simulink model "VVA_pressure_dynamic_basefreq_sin"  (R2023b)
settings: Solver=FixedStepAuto  StartTime=0.0  StopTime=6  MaxStep=1e-3  RelTol=1e-3
values from neighbouring files (symbols this model uses):
  x = [2*10^5	3*10^5	4*10^5	5*10^5	6*10^5	7*10^5	8*10^5]    [Q.m]    (also in new_run_compare_export_jieyue.m = ts.Data(:); new_run_compare_sin_export.m = ts.Data(:); objfun_ga.m = double(x(:)); run_compare_jieyue.m = ts.Data(:))
  y = [0 ... (first row only)    [Q.m]    (also in new_run_compare_export_jieyue.m = interp1(t0u, x0u, t(:), method, 'extrap'); new_run_compare_sin_export.m = interp1(t0u, x0u, t(:), method, 'extrap'); objfun_ga.m = y(ia); run_compare_jieyue.m = interp1(t0u, x0u, t(:), method, 'extrap'))
  z = [0.893557423	1.334431826	1.76701406	2.210901891	2.65062	3.098039216	3.535707573 ... (first row only)    [Q.m]
undefined symbols (not defined in the file or in its folder): freq_mode
libraries: fuzblock x2, simulink x2
settings Model: Creator=Administrator  LastModifiedBy=47371
settings SolverCC: MaxConsecutiveMinStep=2  ZeroCrossAlgorithm=Adaptive  AlgebraicLoopSolver=TrustRegion
settings DebuggingCC: MaskedZcDiagnostic=none  IgnoredZcDiagnostic=none  ArithmeticOperatorsInVariantConditions=warning
settings SFSimCC: CustomCodeUndefinedFunction=UseInterfaceOnly

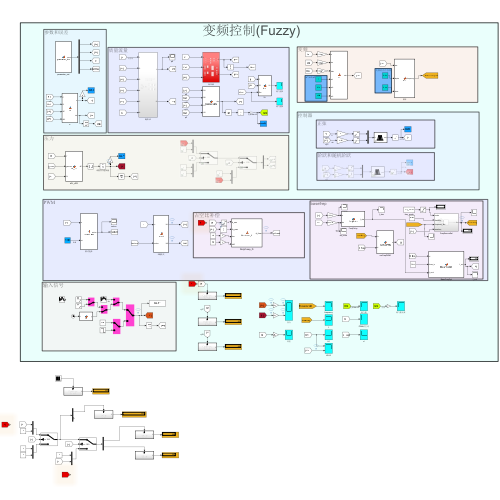
[thumbnail: Simulink's stored preview of the top-level diagram]
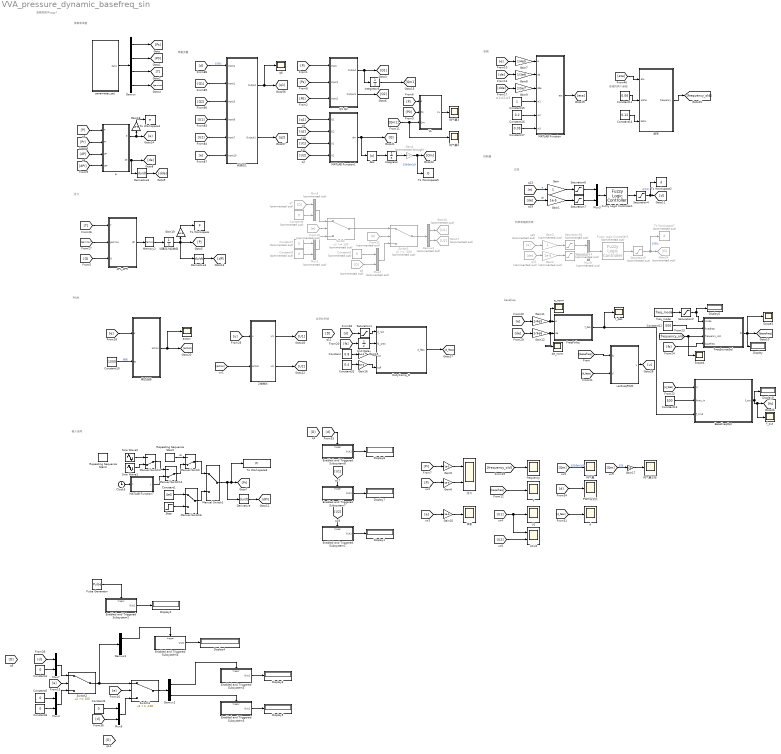
== system VVA_pressure_dynamic_basefreq_sin ==
  note: 输入信号
  note: 占空比补偿
  note: 正弦
  note: 阶跃和随机阶跃
  note: 变频控制(Fuzzy)
  note: 变频
  note: basefrep
  note: 控制器
  note: 压力
  note: 参数和误差
  note: 质量流量
  note: PWM
  note: 变频的两个参数
  note: w1,w2,w3
  2阀模式 : MATLAB Function  TreatAsAtomicUnit=on  SystemSampleTime=0.001
  Abs : Abs  SaturateOnIntegerOverflow=off
  BaseFreqOpt : MATLAB Function  TreatAsAtomicUnit=on
  Clock5 : Clock
  Constant : Constant  Value=0.8
  Constant1 : Constant  Value=4e5
  Constant10 : Constant  Value=1000
  Constant11 : Constant  Value=0.06
  Constant12 : Constant  Value=500
  Constant13 : Constant  Value=500
  Constant14 : Constant  Value=0.12
  Constant15 : Constant
  Constant16 : Constant  Value=0.2
  Constant17 : Constant  Value=0.05
  Constant{2,4..5,8} (4 alike) : Constant  Value=0
  Constant{3,6..7,9} (4 alike) : Constant  Commented=on  Value=0
  Constant32 : Constant  Value=0.4
  Demux : Demux
  Demux1 : Demux  Commented=on  Outputs=2
  Demux2 : Demux  Outputs=2
  Demux3 : Demux  Outputs=2
  Derivative : Derivative
  Derivative1 : Derivative
  Derivative2 : Derivative
  Display{,1..9} (10 alike) : Display
  DutyComp_D : MATLAB Function  TreatAsAtomicUnit=on
  Enabled and Triggered Subsystem1 : Subsystem  TreatAsAtomicUnit=on
  Enabled and Triggered Subsystem2 : Subsystem  TreatAsAtomicUnit=on
  Enabled and Triggered Subsystem3 : Subsystem  TreatAsAtomicUnit=on
  Enabled and Triggered Subsystem4 : Subsystem  TreatAsAtomicUnit=on
  Enabled and Triggered Subsystem5 : Subsystem  TreatAsAtomicUnit=on
  Enabled and Triggered Subsystem7 : Subsystem  TreatAsAtomicUnit=on
  Enabled and Triggered Subsystem8 : Subsystem  TreatAsAtomicUnit=on
  FreqPolicy : MATLAB Function  TreatAsAtomicUnit=on
  FreqSourceSel : Subsystem
  From14 : From  Commented=on  GotoTag=e
  From32 : From  Commented=on  GotoTag=e
  Fuzzy Logic Controller1 : fuzblock/Fuzzy Logic  Controller  FIS="\"fuzzy_pressure_516.fis\""  OutputSampleNumber=101  DataType=double  FuzzifiedInputs=off  RuleFiringStrengths=off  RuleOutputs=off  AggregatedOutputs=off  SimulateUsing=Interpreted execution  OutOfRangeInputValueMessage=warning  NoRuleFiredMessage=warning  EmptyOutputFuzzySetMessage=warning
  Fuzzy Logic Controller3 : fuzblock/Fuzzy Logic  Controller  Commented=on  FIS="\"fuzzy_pressure_516.fis\""  OutputSampleNumber=101  DataType=double  FuzzifiedInputs=off  RuleFiringStrengths=off  RuleOutputs=off  AggregatedOutputs=off  SimulateUsing=Interpreted execution  OutOfRangeInputValueMessage=warning  NoRuleFiredMessage=warning  EmptyOutputFuzzySetMessage=warning
  Gain : Gain
  Gain{1,5..6,10,18..19} (6 alike) : Gain  Gain=1e-5
  Gain11 : Gain  Gain=1/4e5
  Gain12 : Gain  Gain=1/3e6
  Gain15 : Gain  Gain=1e-3
  Gain16 : Gain  Gain=1e-3
  Gain17 : Gain  Gain=1/3
  Gain2 : Gain  Commented=on  Gain=1e-5
  Gain3 : Gain  Commented=on
  Gain4 : Gain  Commented=through  Gain=1/3
  Gain7 : Gain  Gain=1/4e5
  Gain8 : Gain  Gain=1/3e6
  Gain9 : Gain  Gain=1/5e7
  Goto16 : Goto  Commented=on  GotoTag=U1
  Goto17 : Goto  Commented=on  GotoTag=U2
  Goto24 : Goto  Commented=on  GotoTag=D
  Integrator : Integrator
  Integrator3 : Integrator
  MATLAB Function : MATLAB Function  TreatAsAtomicUnit=on
  MATLAB Function1 : MATLAB Function  TreatAsAtomicUnit=on
  MATLAB Function7 : MATLAB Function  TreatAsAtomicUnit=on
  Manual Switch : ManualSwitch  CurrentSetting=0
  Manual Switch1 : ManualSwitch
  Manual Switch14 : ManualSwitch  CurrentSetting=0
  Manual Switch3 : ManualSwitch  CurrentSetting=0
  Manual Switch6 : ManualSwitch
  Memory2 : Memory  InitialCondition=10
  Mux{1..2,5,9} (4 alike) : Mux  Commented=on  Inputs=2
  Mux{3..4,6..7} (4 alike) : Mux  Inputs=2
  PWM占空比 : Scope
  Pulse Generator : DiscretePulseGenerator  PulseType=Time based  Period=0.01  PulseWidth=5
  Q1 Q2 : Subsystem
  Repeating Sequence Stair2 : simulink/Sources/Repeating Sequence Stair  OutValues=[1.01325e5 4e5 3e5 6e5 3.5e5 5e5 4.5e5 2e5].'  tsamp=1  OutMin=[]  OutMax=[]  OutDataTypeStr=double  OutputDataTypeScalingMode=double  OutDataType=fixdt(0,8)  ConRadixGroup=Best Precision: Vector-wise  OutScaling=2^-12
  Repeating Sequence Stair3 : simulink/Sources/Repeating Sequence Stair  OutValues=[1.01325e5 3e5 2e5 5e5 4e5 2.5e5 1.01325e5].'  tsamp=1  OutMin=[]  OutMax=[]  OutDataTypeStr=double  OutputDataTypeScalingMode=double  OutDataType=fixdt(0,8)  ConRadixGroup=Best Precision: Vector-wise  OutScaling=2^-12
  Saturation1 : Saturate  UpperLimit=1  LowerLimit=0
  Saturation10 : Saturate  Commented=on  UpperLimit=4  LowerLimit=-4
  Saturation11 : Saturate  Commented=on  UpperLimit=35  LowerLimit=-35
  Saturation2 : Saturate  UpperLimit=3  LowerLimit=1
  Saturation4 : Saturate  UpperLimit=0.98  LowerLimit=0.1
  Saturation6 : Saturate  UpperLimit=4  LowerLimit=-4
  Saturation7 : Saturate  UpperLimit=35  LowerLimit=-35
  Saturation9 : Saturate  Commented=on  UpperLimit=0.98  LowerLimit=0.1
  Scope3 : Scope
  Scope4 : Scope
  Sine Wave1 : Sin  Amplitude=2.98675e5  Bias=4e5  Frequency=2*pi*0.25  SampleTime=0
  Sine Wave2 : Sin  Amplitude=2.98675e5  Bias=4e5  Frequency=2*pi*0.5  SampleTime=0
  Step : Step  Before=6e5  After=3e5  SampleTime=0
  Switch : Switch  Commented=on  Threshold=100  SaturateOnIntegerOverflow=off  InputSameDT=off
  Switch1 : Switch  Commented=on  Threshold=-100  SaturateOnIntegerOverflow=off  InputSameDT=off
  Switch2 : Switch  Threshold=100  SaturateOnIntegerOverflow=off  InputSameDT=off
  Switch3 : Switch  Threshold=-100  SaturateOnIntegerOverflow=off  InputSameDT=off
  To Workspace : ToWorkspace  VariableName=P  SaveFormat=Timeseries  SampleTime=0.003
  To Workspace1 : ToWorkspace  VariableName=e  SaveFormat=Timeseries  SampleTime=0.003
  To Workspace2 : ToWorkspace  VariableName=d  SaveFormat=Timeseries  SampleTime=0.003
  To Workspace3 : ToWorkspace  VariableName=Pr  SaveFormat=Timeseries  SampleTime=-1
  To Workspace5 : ToWorkspace  VariableName=Q  SaveFormat=Timeseries  SampleTime=0.003
  To Workspace7 : ToWorkspace  Commented=on  VariableName=d  SaveFormat=Timeseries  SampleTime=0.003
  U1 : Scope
  "U1U2 " : Scope  NumInputPorts=2
  Unit Delay : UnitDelay  SampleTime=-1  HasFrameUpgradeWarning=on
  VL : MATLAB Function  TreatAsAtomicUnit=on
  action : Scope
  d : Scope
  dPL_dPR : MATLAB Function  TreatAsAtomicUnit=on
  de_norm : Scope
  e : MATLAB Function  TreatAsAtomicUnit=on
  e_norm : Scope
  f : Scope
  f_des : Scope
  f_out : Scope
  freq_mode : Constant  Value=freq_mode  SampleTime=-1
  frequency : Scope
  parameter_set : MATLAB Function  TreatAsAtomicUnit=on
  q30 : From  Commented=on  GotoTag=e
  q31 : From  Commented=on  GotoTag=de
  q6 : Scope
  q7 : From  Commented=on  GotoTag=D
  q8 : From  Commented=on  GotoTag=D
  varFreqPWM : MATLAB Function  TreatAsAtomicUnit=on
  压力 : Scope  NumInputPorts=2
  模式选择 : MATLAB Function  TreatAsAtomicUnit=on  SystemSampleTime=0.001
  耗气量 : Scope
  耗气量2 : Scope
  耗气量3 : Scope
  耗气量正弦 : Scope
  设置压力起始值 : Integrator  InitialCondition=1.01325e5
  误差 : Scope
  阀滞后1 : Subsystem
  频率 : MATLAB Function  TreatAsAtomicUnit=on
  wires:
  parameter_set/1(para) -> Demux/1
  Demux/1 -> [Ps]
  Demux/2 -> [P0]
  Demux/3 -> [T]
  Demux/4 -> [gamma]
  dPL_dPR/1(dP) -> Memory2/1
  设置压力起始值/1 -> Gain19/1, [P], Derivative1/1
  [gamma] -> dPL_dPR/2(gamma)
  [T] -> dPL_dPR/1(T)
  [Q] -> dPL_dPR/3(Q)
  [P] -> e/1(P)
  Memory2/1 -> 设置压力起始值/1
  MATLAB Function1/1(dm) -> Abs/1, [Q]
  [Ps] -> Q1 Q2/2(Input1)
  [P0] -> Q1 Q2/3(Input2)
  [P] -> Q1 Q2/1(Input)
  Q1 Q2/1(Output) -> Integrator3/1, [Q1]
  Q1 Q2/2(Output1) -> [Q2]
  [d] -> 阀滞后1/1(Input1)  "占空比"
  [Q1] -> 阀滞后1/2(Input2)
  阀滞后1/1(Output) -> q6/1, [q1]
  阀滞后1/2(Output1) -> [q2]
  [e] -> 阀滞后1/6(Input10)
  [U1] -> 阀滞后1/4(Input6)
  [U2] -> 阀滞后1/5(Input7)
  [Q2] -> 阀滞后1/3(Input3)
  [q1] -> MATLAB Function1/1(Q1)
  [q2] -> MATLAB Function1/2(Q2)
  [U2] -> MATLAB Function1/4(U2)
  [Pr] -> e/2(Pr)
  [dPr] -> e/4(dPr)
  [dP] -> e/3(dP)
  e/1(e) -> Gain18/1, [e]
  e/2(de) -> Derivative2/1, [de]
  Derivative1/1 -> [dP]
  Demux1/2 -> Goto17/1
  Mux5/1 -> Switch/1
  From14/1 -> Switch/2
  Constant6/1 -> Mux5/2
  Constant3/1 -> Mux2/1
  MATLAB Function/1(eta) -> [eta]
  Constant14/1 -> 频率/3(beta)
  Constant17/1 -> MATLAB Function/6(w3)
  Constant15/1 -> MATLAB Function/4(w1)
  频率/1(frequency) -> [frequency_old]
  [eta] -> 频率/1(eta)
  Constant16/1 -> MATLAB Function/5(w2)
  Constant11/1 -> 频率/2(alpha)
  Derivative2/1 -> [dde]
  Mux3/1 -> Fuzzy Logic Controller1/1
  [e] -> Gain/1  "e"
  [de] -> Gain1/1  "de"
  Fuzzy Logic Controller1/1 -> Saturation4/1
  Saturation4/1 -> To Workspace2/1, [d]  "占空比"
  q7/1 -> Mux5/1
  q8/1 -> Mux2/2
  Switch1/1 -> Demux1/1
  From32/1 -> Switch1/2
  Constant7/1 -> Mux1/1
  Constant9/1 -> Mux1/2
  Mux1/1 -> Switch/3
  Switch/1 -> Switch1/1
  Mux2/1 -> Switch1/3
  Saturation6/1 -> Mux3/1
  Saturation7/1 -> Mux3/2
  Gain/1 -> Saturation6/1
  Gain1/1 -> Saturation7/1
  q31/1 -> Gain2/1
  q30/1 -> Gain3/1
  Saturation11/1 -> Mux9/2
  Saturation10/1 -> Mux9/1
  Fuzzy Logic Controller3/1 -> Saturation9/1
  Mux9/1 -> Fuzzy Logic Controller3/1
  Gain2/1 -> Saturation11/1
  Gain3/1 -> Saturation10/1
  Abs/1 -> Integrator/1
  Integrator/1 -> Gain4/1
  Gain4/1 -> To Workspace5/1, [Qm]  "正弦Gain1/3"
  Constant/1 -> Gain15/1
  Constant32/1 -> Gain16/1
  Gain15/1 -> DutyComp_D/3(ton)
  Gain16/1 -> DutyComp_D/4(toff)
  Integrator3/1 -> [Qm1]
  [P0] -> VL/2(P0)
  [Qm1] -> 耗气量2/1, VL/3(Qm)
  VL/1(VL) -> 耗气量3/1
  [P] -> VL/1(P)
  Demux1/1 -> Goto16/1
  Enabled and Triggered Subsystem3/1(Out1) -> Display3/1
  Demux2/1 -> Enabled and Triggered Subsystem3/Trigger
  Mux6/1 -> Switch3/3
  Switch2/1 -> Demux3/1, Switch3/1
  Mux4/1 -> Switch2/3
  Constant8/1 -> Mux4/2
  Constant5/1 -> Mux4/1
  [e] -> Switch3/2
  Switch3/1 -> Demux2/1
  Constant2/1 -> Mux6/1
  Constant4/1 -> Mux7/2
  [e] -> Switch2/2
  Mux7/1 -> Switch2/1
  Demux2/2 -> Enabled and Triggered Subsystem5/Trigger
  Demux3/1 -> Enabled and Triggered Subsystem4/Trigger
  Enabled and Triggered Subsystem4/1(Out1) -> Display4/1
  Enabled and Triggered Subsystem5/1(Out1) -> Display5/1
  [U1] -> MATLAB Function1/3(U1)
  模式选择/1(action) -> action/1, [action]
  2阀模式/1(U1) -> [U1]
  2阀模式/2(U2) -> [U2]
  [e] -> 模式选择/1(e)
  [action] -> 2阀模式/2(action)
  Enabled and Triggered Subsystem7/1(Out1) -> Display7/1
  Enabled and Triggered Subsystem8/1(Out1) -> Display8/1
  [U2] -> Enabled and Triggered Subsystem1/Trigger
  Enabled and Triggered Subsystem1/1(Out1) -> Display1/1
  Constant10/1 -> 模式选择/2(et)  "参数"
  [U1] -> Enabled and Triggered Subsystem7/Trigger
  Gain5/1 -> 压力/1
  [Pr] -> Gain5/1
  [P] -> Gain6/1
  Gain6/1 -> 压力/2
  Gain10/1 -> 误差/1
  [e] -> Gain10/1
  [frequency_old] -> frequency/1
  [Qm] -> 耗气量/1  "正弦Gain1/3"
  Saturation9/1 -> Goto24/1, To Workspace7/1  "占空比"
  [U1] -> "U1U2 "/1, U1/1
  [U2] -> "U1U2 "/2
  [d] -> PWM占空比/1
  [Qm] -> Gain17/1  "正弦"
  Gain17/1 -> 耗气量正弦/1
  Gain18/1 -> To Workspace1/1
  Gain19/1 -> To Workspace/1
  Repeating Sequence Stair2/1 -> Manual Switch/1  "8s"
  Manual Switch1/1 -> Derivative/1, To Workspace3/1, [Pr]
  Derivative/1 -> [dPr]
  Manual Switch/1 -> Manual Switch1/1
  Constant1/1 -> Manual Switch6/1
  Manual Switch3/1 -> Manual Switch14/1
  Manual Switch6/1 -> Manual Switch1/2
  MATLAB Function7/1(y) -> Manual Switch14/2
  Step/1 -> Manual Switch6/2
  Sine Wave2/1 -> Manual Switch3/1
  Manual Switch14/1 -> Manual Switch/2
  Clock5/1 -> MATLAB Function7/1(t)
  Sine Wave1/1 -> Manual Switch3/2
  Pulse Generator/1 -> Enabled and Triggered Subsystem2/Trigger
  Enabled and Triggered Subsystem2/1(Out1) -> Display2/1
  BaseFreqOpt/1(f_out) -> f_out/1, [fs], Display9/1
  Saturation1/1 -> DutyComp_D/1(d_raw)
  [frequency_old] -> Scope4/1, FreqSourceSel/3(frequency_old)
  Constant12/1 -> FreqSourceSel/2(fixedfrep)
  freq_mode/1 -> Saturation2/1
  Saturation2/1 -> FreqSourceSel/1(mode), Display6/1
  FreqSourceSel/1(fs) -> Scope3/1, [basefreq], Display/1
  [basefreq] -> varFreqPWM/1(fs)
  Constant13/1 -> BaseFreqOpt/2(fmax_in)
  [e] -> Gain7/1
  Gain7/1 -> MATLAB Function/1(e)
  [de] -> Gain8/1
  Gain8/1 -> MATLAB Function/2(de)
  Gain9/1 -> MATLAB Function/3(dde)
  [dde] -> Gain9/1
  FreqPolicy/1(f_des) -> BaseFreqOpt/3(f_cmd), f_des/1
  DutyComp_D/1(d_feas) -> [d_feas]
  [d_feas] -> varFreqPWM/2(d)
  [d_feas] -> BaseFreqOpt/1(d)
  [fs] -> FreqSourceSel/4(basefreq)
  Unit Delay/1 -> DutyComp_D/2(fs_prev)
  [d] -> Saturation1/1
  varFreqPWM/1(u) -> [u]
  [u] -> 2阀模式/1(u)
  [d_feas] -> d/1
  [basefreq] -> f/1
  [e] -> Gain11/1
  Gain11/1 -> e_norm/1, FreqPolicy/1(e)
  [de] -> Gain12/1
  [fs] -> Unit Delay/1
  Gain12/1 -> de_norm/1, FreqPolicy/2(de)
  [d] -> Enabled and Triggered Subsystem8/Trigger
  [d] -> Mux7/1
  [d] -> Mux6/2

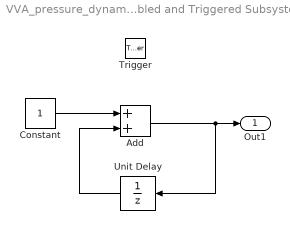
== system VVA_pressure_dynamic_basefreq_sin/Enabled and Triggered Subsystem1 ==
  Trigger : TriggerPort  VariantControl=(inherit)
  Add : Sum
  Constant : Constant
  Unit Delay : UnitDelay  SampleTime=-1  HasFrameUpgradeWarning=on
  Out1 : Outport
  wires:
  Unit Delay/1 -> Add/2
  Add/1 -> Out1/1, Unit Delay/1
  Constant/1 -> Add/1

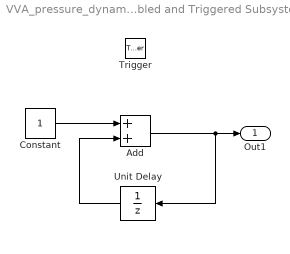
== system VVA_pressure_dynamic_basefreq_sin/Enabled and Triggered Subsystem2 ==
  Trigger : TriggerPort  VariantControl=(inherit)
  Add : Sum
  Constant : Constant
  Unit Delay : UnitDelay  SampleTime=-1  HasFrameUpgradeWarning=on
  Out1 : Outport
  wires:
  Unit Delay/1 -> Add/2
  Add/1 -> Out1/1, Unit Delay/1
  Constant/1 -> Add/1

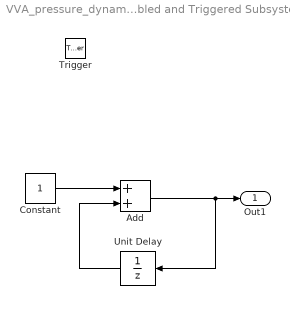
== system VVA_pressure_dynamic_basefreq_sin/Enabled and Triggered Subsystem3 ==
  Trigger : TriggerPort  VariantControl=(inherit)
  Add : Sum
  Constant : Constant
  Unit Delay : UnitDelay  SampleTime=-1  HasFrameUpgradeWarning=on
  Out1 : Outport
  wires:
  Unit Delay/1 -> Add/2
  Add/1 -> Out1/1, Unit Delay/1
  Constant/1 -> Add/1

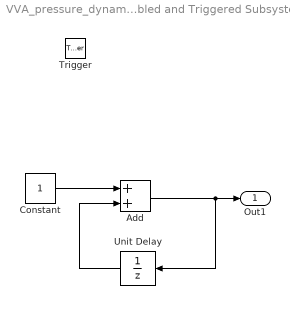
== system VVA_pressure_dynamic_basefreq_sin/Enabled and Triggered Subsystem4 ==
  Trigger : TriggerPort  VariantControl=(inherit)
  Add : Sum
  Constant : Constant
  Unit Delay : UnitDelay  SampleTime=-1  HasFrameUpgradeWarning=on
  Out1 : Outport
  wires:
  Unit Delay/1 -> Add/2
  Add/1 -> Out1/1, Unit Delay/1
  Constant/1 -> Add/1

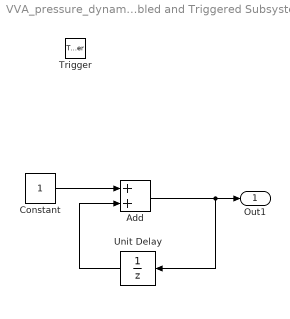
== system VVA_pressure_dynamic_basefreq_sin/Enabled and Triggered Subsystem5 ==
  Trigger : TriggerPort  VariantControl=(inherit)
  Add : Sum
  Constant : Constant
  Unit Delay : UnitDelay  SampleTime=-1  HasFrameUpgradeWarning=on
  Out1 : Outport
  wires:
  Unit Delay/1 -> Add/2
  Add/1 -> Out1/1, Unit Delay/1
  Constant/1 -> Add/1

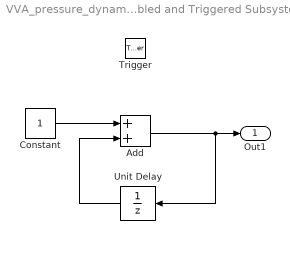
== system VVA_pressure_dynamic_basefreq_sin/Enabled and Triggered Subsystem7 ==
  Trigger : TriggerPort  VariantControl=(inherit)
  Add : Sum
  Constant : Constant
  Unit Delay : UnitDelay  SampleTime=-1  HasFrameUpgradeWarning=on
  Out1 : Outport
  wires:
  Constant/1 -> Add/1
  Add/1 -> Unit Delay/1, Out1/1
  Unit Delay/1 -> Add/2

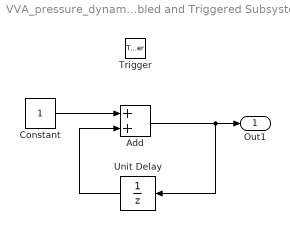
== system VVA_pressure_dynamic_basefreq_sin/Enabled and Triggered Subsystem8 ==
  Trigger : TriggerPort  VariantControl=(inherit)
  Add : Sum
  Constant : Constant
  Unit Delay : UnitDelay  SampleTime=-1  HasFrameUpgradeWarning=on
  Out1 : Outport
  wires:
  Unit Delay/1 -> Add/2
  Add/1 -> Out1/1, Unit Delay/1
  Constant/1 -> Add/1

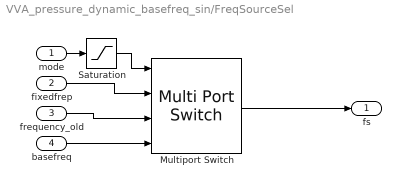
== system VVA_pressure_dynamic_basefreq_sin/FreqSourceSel ==
  mode : Inport
  fixedfrep : Inport  Port=2
  frequency_old : Inport  Port=3
  basefreq : Inport  Port=4
  Multiport Switch : MultiPortSwitch  SaturateOnIntegerOverflow=off  InputSameDT=off
  Saturation : Saturate  UpperLimit=3  LowerLimit=1
  fs : Outport
  wires:
  Multiport Switch/1 -> fs/1
  Saturation/1 -> Multiport Switch/1
  mode/1 -> Saturation/1
  fixedfrep/1 -> Multiport Switch/2
  frequency_old/1 -> Multiport Switch/3
  basefreq/1 -> Multiport Switch/4

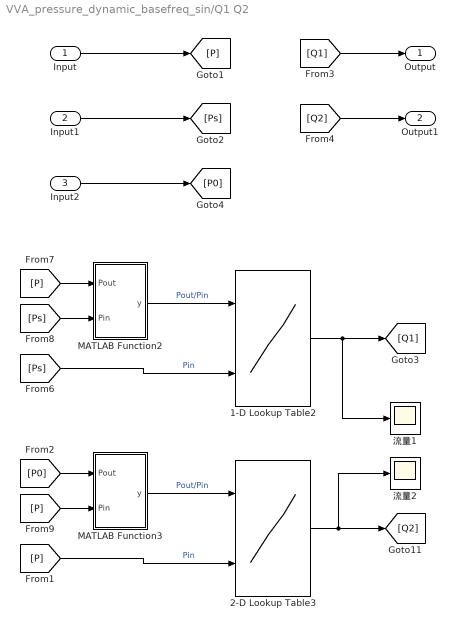
== system VVA_pressure_dynamic_basefreq_sin/Q1 Q2 ==
  Input : Inport
  Input1 : Inport  Port=2
  Input2 : Inport  Port=3
  1-D Lookup Table2 : Lookup_n-D  BreakpointsForDimension1=y  BreakpointsForDimension2=x  Table=z  InterpMethod=Cubic spline  ExtrapMethod=Cubic spline  InternalRulePriority=Speed  RndMeth=Simplest
      settings: InputPortMap=u0,u1
  2-D Lookup Table3 : Lookup_n-D  BreakpointsForDimension1=y  BreakpointsForDimension2=x  Table=z  InterpMethod=Cubic spline  ExtrapMethod=Cubic spline  InternalRulePriority=Speed  RndMeth=Simplest
      settings: InputPortMap=u0,u1
  MATLAB Function2 : MATLAB Function  TreatAsAtomicUnit=on
  MATLAB Function3 : MATLAB Function  TreatAsAtomicUnit=on
  流量1 : Scope
  流量2 : Scope
  Output : Outport
  Output1 : Outport  Port=2
  wires:
  2-D Lookup Table3/1 -> 流量2/1, [Q2]
  [P] -> MATLAB Function2/1(Pout)
  [P0] -> MATLAB Function3/1(Pout)
  MATLAB Function2/1(y) -> 1-D Lookup Table2/1  "Pout/Pin"
  MATLAB Function3/1(y) -> 2-D Lookup Table3/1  "Pout/Pin"
  1-D Lookup Table2/1 -> 流量1/1, [Q1]
  [P] -> MATLAB Function3/2(Pin)
  [Ps] -> MATLAB Function2/2(Pin)
  Input/1 -> [P]
  Input1/1 -> [Ps]
  Input2/1 -> [P0]
  [Q1] -> Output/1
  [Q2] -> Output1/1
  [P] -> 2-D Lookup Table3/2  "Pin"
  [Ps] -> 1-D Lookup Table2/2  "Pin"

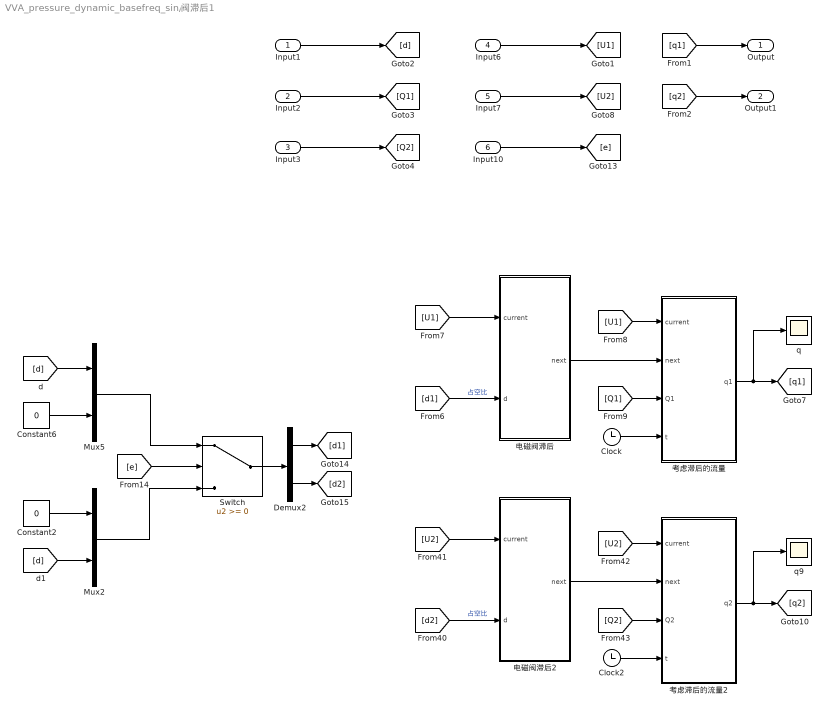
== system VVA_pressure_dynamic_basefreq_sin/阀滞后1 ==
  Input1 : Inport
  Input2 : Inport  Port=2
  Input3 : Inport  Port=3
  Input6 : Inport  Port=4
  Input7 : Inport  Port=5
  Input10 : Inport  Port=6
  " 电磁阀滞后" : MATLAB Function  TreatAsAtomicUnit=on
  " 电磁阀滞后2" : MATLAB Function  TreatAsAtomicUnit=on
  Clock : Clock
  Clock2 : Clock
  Constant2 : Constant  Value=0
  Constant6 : Constant  Value=0
  Demux2 : Demux  Outputs=2
  Mux2 : Mux  Inputs=2
  Mux5 : Mux  Inputs=2
  Switch : Switch  SaturateOnIntegerOverflow=off  InputSameDT=off
  q : Scope
  q9 : Scope
  考虑滞后的流量 : MATLAB Function  TreatAsAtomicUnit=on
  考虑滞后的流量2 : MATLAB Function  TreatAsAtomicUnit=on
  Output : Outport
  Output1 : Outport  Port=2
  wires:
  Clock2/1 -> 考虑滞后的流量2/4(t)
  [U1] -> " 电磁阀滞后"/1(current)
  Clock/1 -> 考虑滞后的流量/4(t)
  [Q1] -> 考虑滞后的流量/3(Q1)
  [d1] -> " 电磁阀滞后"/2(d)  "占空比"
  考虑滞后的流量/1(q1) -> q/1, [q1]
  " 电磁阀滞后"/1(next) -> 考虑滞后的流量/2(next)
  [Q2] -> 考虑滞后的流量2/3(Q2)
  [U1] -> 考虑滞后的流量/1(current)
  考虑滞后的流量2/1(q2) -> [q2], q9/1
  [U2] -> " 电磁阀滞后2"/1(current)
  [d2] -> " 电磁阀滞后2"/2(d)  "占空比"
  " 电磁阀滞后2"/1(next) -> 考虑滞后的流量2/2(next)
  [U2] -> 考虑滞后的流量2/1(current)
  Input1/1 -> [d]
  Input3/1 -> [Q2]
  Input2/1 -> [Q1]
  [q1] -> Output/1
  [q2] -> Output1/1
  Input7/1 -> [U2]
  Input6/1 -> [U1]
  Input10/1 -> [e]
  Mux2/1 -> Switch/3
  Mux5/1 -> Switch/1
  Constant6/1 -> Mux5/2
  [d] -> Mux2/2
  Demux2/1 -> [d1]
  Switch/1 -> Demux2/1
  Constant2/1 -> Mux2/1
  [e] -> Switch/2
  [d] -> Mux5/1
  Demux2/2 -> [d2]

== matlab function VVA_pressure_dynamic_basefreq_sin/BaseFreqOpt ==
  settings: updateMethod=DISCRETE
  data: d input; f_out output; fmax_in input; f_cmd input
function f_out = BaseFreqOpt(d, fmax_in, f_cmd) %#codegen
% PWM基础频率动态优化：物理可行域上限 + 高频预算 + 平滑 + 斜率限制
% 输入:
%   d       : 占空比(0..1)
%   fmax_in : 外部硬上限(Hz)，通常给500
%   f_cmd   : 期望频率(Hz)，来自 FreqPolicy 或 freq门控
% 输出:
%   f_out   : 最终基础频率(Hz)

% ====== 参数区（按你模型需要微调） ======
Ts = 1e-4;          % 必须与 Solver Fixed-step 一致

% 阀运动约束（与你模型一致）
ton  = 0.0008;      % 总开时间(s)
toff = 0.0004;      % 总关时间(s)

kf = 0.94;          % 安全系数(0~1)，越小越保守
f_min = 60;         % 最低频率(Hz)：太低会慢/不稳
f_mid = 160;        % 预算超限时压回的“中频”(Hz)

% 平滑 & 斜率限制
lambda_lp = 0.97;   % 低通滤波(0.90~0.98). 越大越慢越平滑
ramp_up   = 3000;   % 上升最大斜率(Hz/s)
ramp_down = 20000;   % 下降最大斜率(Hz/s)（不要无限快，避免周期突变）

% 高频预算（用来压 nsw：允许短时高频burst，禁止长期高频）
S_max = 40;         % 预算阈值（越小越省开关；过小会影响RMSE）
leak  = 80;         % 预算泄放速度（越大恢复越快）

% ====== 强制标量 & 防御 ======
d      = d(1);
fmax_in = fmax_in(1);
f_cmd  = f_cmd(1);

d = min(max(d,0.0),1.0);
fmax_in = max(fmax_in, 1.0);
f_cmd   = max(f_cmd  , 1.0);

% ====== 物理可行上限：保证 d*T>=ton 且 (1-d)*T>=toff ======
% T = 1/f, 所以 f <= d/ton 且 f <= (1-d)/toff
if (d <= 1e-6) || (d >= 1-1e-6)
    f_upper_phy = f_min; % 极端占空比直接回落到最低可行
else
    f1 = d/max(ton,1e-12);
    f2 = (1-d)/max(toff,1e-12);
    f_upper_phy = kf * min(f1, f2);
end

% 与外部上限合并
f_upper = min(f_upper_phy, fmax_in);
f_lower = min(f_min, f_upper);   % 防止下限>上限

% ====== 目标频率（先限幅） ======
f_tgt = min(max(f_cmd, f_lower), f_upper);

% ====== 高频预算器：抑制长期高频 ======
persistent S f_prev
if isempty(S);      S = 0;      end
if isempty(f_prev); f_prev = f_tgt; end

% 预算累积：高于 f_lower 的部分计入开关“成本”
S = S + max(f_prev - f_mid, 0) * Ts;
% 预算泄放：让系统回到低频后逐渐“恢复额度”
S = max(0, S - leak*Ts);

if S > S_max
    f_tgt = min(f_tgt, f_mid);
end

% ====== 平滑（低通） ======
f_lp = lambda_lp * f_prev + (1 - lambda_lp) * f_tgt;

% ====== 斜率限制（上升慢、下降也有限制避免突变） ======
df = f_lp - f_prev;
df = min(df,  ramp_up  * Ts);
df = max(df, -ramp_down* Ts);
f_out = f_prev + df;

% 最终限幅
f_out = min(max(f_out, f_lower), f_upper);

% 更新记忆
f_prev = f_out;
end

== matlab function VVA_pressure_dynamic_basefreq_sin/MATLAB Function ==
  data: e input; eta output; de input; dde input; w1 input; w2 input; w3 input
function eta = fcn(e,de,dde,w1,w2,w3)   % w1,w2,w3 三个参数 具体大小怎么确定

%w1=1;        %三个参数w1,w2,w3
%w2=0.5;
%w3=1;

eta = w1*e+w2*de+w3*dde;
eta = max(min(eta, 0.5), -0.5);   % 把η夹到[-0.5,0.5]

== matlab function VVA_pressure_dynamic_basefreq_sin/varFreqPWM ==
  settings: updateMethod=DISCRETE
  data: fs input; u output; d input
function u = VarFreqPWM(fs, d) %#codegen
% 可变频PWM（相位累积法）
Ts = 1e-4;  % 与模型 fixed-step 一致

persistent phi
if isempty(phi)
    phi = 0;  % 相位 in [0,1)
end

% 防御
fs = fs(1);
d  = d(1);

fs = max(fs, 1.0);
fs = min(fs, 1e5);
d  = min(max(d,0.0),1.0);

% 相位累积（每步前进 fs*Ts，超过1回绕）
phi = phi + fs*Ts;
phi = phi - floor(phi);

% PWM：phi < d -> 高电平
u = double(phi < d);
end

== matlab function VVA_pressure_dynamic_basefreq_sin/parameter_set ==
  data: para output
function para = parameter_set()  %parameter 变量
global t0_1 t0_2 t0_3 t0_4 flag1 flag2 flag3 flag4;
para = 1:4;  

Ps = 8e5;
P0 = 1.01325e5;
T=  293.15;
gamma =1.4;                



para(1) = Ps;           
para(2) = P0;
para(3) = T;
para(4) = gamma;

== matlab function VVA_pressure_dynamic_basefreq_sin/FreqPolicy ==
  settings: updateMethod=DISCRETE
  data: e input; f_des output; de input
function f_des = FreqPolicy(e, de) %#codegen
% 目标：大误差低频；中误差中频；小误差默认中/低频；
%      只有在“超调风险/卡住(stall)”时短时 burst 到高频；
%      误差很小且变化很慢 -> 进入 hold，强制降到 f_hold。

Ts = 1e-4;  % 必须与你模型 fixed-step 一致

%% ===== 频率档位 =====
f_hold = 120;     % 稳态保持频率（越低越省开关，但太低可能更易抖/泄漏）
f_low  = 90;     % 大误差：低频粗调
f_mid  = 200;    % 中误差：中频
f_high = 450;    % burst：高频精调（注意最终可能被 BaseFreqOpt 的物理上限卡住）

%% ===== 误差阈值（按 e_norm 的量级调）=====
E_hi   = 0.45;   % >E_hi: 低频
E_lo   = 0.18;   % <E_lo: “小误差区”（默认不常驻高频，把高频留给 burst）
E_hold = 0.02;   % 进入稳态判据（越小越严格）

%% ===== de 滤波与稳态判据 =====
Tf_de  = 0.01;                   % de 低通时间常数
a_de   = exp(-Ts/max(Tf_de,1e-12));
D_hold = 0.005;                   % |de| 很小认为"稳态"（按你的 de_norm 量级调）

%% ===== burst 判据 =====
E_risk = 0.06;   % 接近目标
D_risk = 0.03;   % 仍然“冲得很快”才触发 burst（防止零附近一直 burst）
T_burst = 0.03;  % burst 持续时间(s)
N_burst = max(int32(1), int32(T_burst/Ts));

%% ===== stall（卡住）判据：误差不小但 de 很小，给一脚 burst 破静摩擦 =====
D_stall = 0.002;
T_stall = 0.03;
N_stall = max(int32(1), int32(T_stall/Ts));

%% ===== 取标量 =====
e  = e(1);
de = de(1);

%% ===== de 低通 =====
persistent de_f
if isempty(de_f)
    de_f = de;
end
de_f = a_de*de_f + (1-a_de)*de;

E = abs(e);
D = abs(de_f);

%% ===== 稳态 hold 计时：E 很小且 D 很小持续一段时间才进入 =====
persistent hold_cnt
if isempty(hold_cnt)
    hold_cnt = int32(0);
end
N_hold = max(int32(1), int32(0.005/Ts));   % 20ms 连续满足才认为稳态

if (E < E_hold) && (D < D_hold)
    if hold_cnt < N_hold
        hold_cnt = hold_cnt + 1;
    end
else
    hold_cnt = int32(0);
end
in_hold = (hold_cnt >= N_hold);

%% ===== 基础频率（不常驻高频）=====
if E > E_hi
    f_base = f_low;
elseif E > E_lo
    % E 从 E_hi -> E_lo：频率从 low 平滑过渡到 mid
    w = (E - E_lo) / max(E_hi - E_lo, 1e-12);   % 0..1
    f_base = f_mid + (f_low - f_mid)*w;
else
    % 小误差区：默认只给 mid（或你也可以给 low），高频交给 burst
    f_base = f_mid;
end

%% ===== burst：超调风险 or stall =====
persistent burst_cnt stall_cnt
if isempty(burst_cnt), burst_cnt = int32(0); end
if isempty(stall_cnt), stall_cnt = int32(0); end

% 超调风险：误差接近 0 且仍在快速逼近（e*de_f<0 且 |de_f|够大）
risk = (~in_hold) && (E < E_risk) && (e*de_f < 0) && (D > D_risk);

% stall：误差不小但导数极小，持续一段时间
if (E > E_lo) && (D < D_stall)
    if stall_cnt < N_stall
        stall_cnt = stall_cnt + 1;
    end
else
    stall_cnt = int32(0);
end
stall = (stall_cnt >= N_stall);

if in_hold
    burst_cnt = int32(0);  % 稳态不 burst
elseif risk || stall
    burst_cnt = N_burst;
elseif burst_cnt > 0
    burst_cnt = burst_cnt - 1;
end

%% ===== 输出 =====
if in_hold
    f_des = f_hold;
elseif burst_cnt > 0
    f_des = f_high;
else
    f_des = f_base;
end

f_des = max(f_des, 1.0);
end

== matlab function VVA_pressure_dynamic_basefreq_sin/频率 ==
  settings: updateMethod=DISCRETE
  data: frequency output; eta input; alpha input; beta input
function frequency = fcn(eta, alpha, beta) %#codegen
% old: 三档频率 + “高频burst” + 稳态省开关
% 目标：大误差低频粗调；中误差中频；小误差默认低频（省开关）
%      只有在接近目标且可能穿越/超调时，短时提升到高频抑制纹波/超调

% --- 标量化（避免1-D向量传入导致异常） ---
eta   = eta(1);
alpha = alpha(1);
beta  = beta(1);

A = abs(eta);

% --- 参数（你可以先用默认，再微调） ---
f_hi  = 500;
f_mid = 300;
f_lo  = 100;

hys = 0;                 % 滞回（可设 0.002~0.01，视eta尺度）
Ts  = 1e-4;              % 与模型 fixed-step 一致
T_burst = 0.02;          % 高频 burst 时长(秒) 10~50ms
N_burst = max(1, int32(T_burst/Ts));

% “穿越/快速变化”判据阈值：用eta变化率粗略估计
deta_thr = 0.02;         % 视eta尺度调（太小会频繁burst）

% --- 记忆：用于检测穿越/变化率、以及做burst计数 ---
persistent eta_prev burst_cnt f_old
if isempty(eta_prev)
    eta_prev  = eta;
    burst_cnt = int32(0);
    f_old     = f_lo;
end

% 穿越风险/变化率估计（注意先用旧值再更新）
deta  = eta - eta_prev;
cross = (eta * eta_prev < 0);    % 误差变号：可能穿越
eta_prev = eta;

% --- burst触发逻辑：接近目标(小误差)时，如果穿越或变化率大，则短时高频 ---
trigger_burst = (A < alpha - hys) && (cross || abs(deta) > deta_thr);

if burst_cnt > 0
    burst_cnt = burst_cnt - 1;
elseif trigger_burst
    burst_cnt = N_burst;
end

% --- 基础档位选择（省开关口味：小误差默认低频，不默认500） ---
if A >= beta + hys
    f_cmd = f_lo;                 % 大误差：低频粗调
elseif A >= alpha + hys
    f_cmd = f_mid;                % 中误差：中频
else
    f_cmd = f_lo;                 % 小误差：默认低频（关键！防止锁500）
end

% --- burst期间强制高频 ---
if burst_cnt > 0
    f_cmd = f_hi;
end

% --- 频率平滑（可选）：上升慢一点、下降快一点（避免长时间高频） ---
lambda_up = 0.85;                 % 0~0.9，越大越平滑
if f_cmd < f_old
    f_old = f_cmd;                % 下降：立即降（省开关）
else
    f_old = lambda_up*f_old + (1-lambda_up)*f_cmd;  % 上升：慢一点
end

frequency = f_old;
end

== matlab function VVA_pressure_dynamic_basefreq_sin/MATLAB Function7 ==
  data: t input; y output
function y = fcn(t)
%#codegen
P0  = 4e5;     % 偏置(Pa)
A   = 1e5;     % 总幅值尺度(Pa)

% 多频(Hz) —— 0.6s内可观测
f1 = 1;   a1 = 0.6;   ph1 = 0.0;
f2 = 4;   a2 = 0.3;   ph2 = 1.0;
f3 = 12;  a3 = 0.1;   ph3 = -0.7;

y = P0 + A*( ...
    a1*sin(2*pi*f1*t + ph1) + ...
    a2*sin(2*pi*f2*t + ph2) + ...
    a3*sin(2*pi*f3*t + ph3));

% 可选：夹紧，避免参考压力超物理范围
Pmin = 1e5;
Pmax = 4.2e5;
y = min(max(y, Pmin), Pmax);
end

== matlab function VVA_pressure_dynamic_basefreq_sin/DutyComp_D ==
  settings: updateMethod=DISCRETE
  data: d_feas output; d_raw input; fs_prev input; ton input; toff input
function d_feas = DutyComp_D(d_raw, fs_prev, ton, toff) %#codegen
% 把占空比拉回“在当前频率下可实现”的区间：
% d*T >= ton  且 (1-d)*T >= toff

d_raw  = d_raw(1);
fs_prev = fs_prev(1);
ton    = ton(1);
toff   = toff(1);

d_raw = min(max(d_raw,0.0),1.0);
fs_prev = max(fs_prev, 1.0);

T = 1/fs_prev;

d_min = ton / max(T,1e-12);
d_max = 1 - toff / max(T,1e-12);

% 防止不可行区间
d_min = min(max(d_min,0.0),1.0);
d_max = min(max(d_max,0.0),1.0);

if d_min > d_max
    % 极端情况下取中间值
    d_feas = 0.5;
else
    d_feas = min(max(d_raw, d_min), d_max);
end
end

== matlab function VVA_pressure_dynamic_basefreq_sin/阀滞后1/ 电磁阀滞后 ==
  settings: updateMethod=DISCRETE
  data: current input; next output; d input
function next = getNextPWMLevel(current, d)
    % current: 当前PWM信号电平 (0或1)
    % d: 占空比 (0到1之间的值)
    % next: 下一时刻PWM信号电平 (0或1)
    
    if current == 0
        if rand <= d
            next = 1;
        else
            next = 0;
        end
    else
        if rand <= (1 - d)
            next = 0;
        else
            next = 1;
        end
    end
end

== matlab function VVA_pressure_dynamic_basefreq_sin/阀滞后1/ 电磁阀滞后2 ==
  settings: updateMethod=DISCRETE
  data: current input; next output; d input
function next = getNextPWMLevel(current, d)
    % current: 当前PWM信号电平 (0或1)
    % d: 占空比 (0到1之间的值)
    % next: 下一时刻PWM信号电平 (0或1)
    
    if current == 0
        if rand <= d
            next = 1;
        else
            next = 0;
        end
    else
        if rand <= (1 - d)
            next = 0;
        else
            next = 1;
        end
    end
end

== matlab function VVA_pressure_dynamic_basefreq_sin/阀滞后1/考虑滞后的流量 ==
  data: current input; q1 output; next input; Q1 input; t input
function q1= lag(current,next,Q1,t)
period=0.55e-3; %阀开启或关闭时间

mode = 0;
flag1 = 1;

if (current == 0 && next == 0) || (current == 1 && next == 1)
    mode = 0;%不变模式
end
if current == 0 && next == 1
    mode =1;%上升模式
end
if current == 1 && next == 0
    mode =2;%下降模式
end

switch(mode)
    case 0
        q1   = Q1;  %不动模式，流量保持不变
    case 1         %从0到1，流量缓慢增加
        if flag1 == 1
            t0_1 = t;
            flag1 = 0;
        end
        t1 = t - t0_1;
        if t1<=period
            q1 = Q1/period*t1;
        else
            q1 = Q1;
            flag1 = 1;
        end
        
    case 2         %从1到0，流量缓慢减小
        if flag1 == 1
            t0_1 = t;
           flag1 = 0;
        end
        t1 = t - t0_1;
        
        if t1<=period
            q1 = Q1/period*(period - t1);
        else
            q1 = Q1;
            flag1 = 1;
        end
    otherwise
        q1 = Q1;
end

== matlab function VVA_pressure_dynamic_basefreq_sin/阀滞后1/考虑滞后的流量2 ==
  data: current input; q2 output; next input; Q2 input; t input
function q2= lag(current,next,Q2,t)
period=0.55e-3; %阀开启或关闭时间

mode = 0;
flag2 = 1;

if (current == 0 && next == 0) || (current == 1 && next == 1)
    mode = 0;%不变模式
end
if current == 0 && next == 1
    mode =1;%上升模式
end
if current == 1 && next == 0
    mode =2;%下降模式
end

switch(mode)
    case 0
        q2   = Q2;  %不动模式，流量保持不变
    case 1         %从0到1，流量缓慢增加
        if flag2 == 1
            t0_2 = t;
            flag2 = 0;
        end
        t1 = t - t0_2;
        if t1<=period
            q2 = Q2/period*t1;
        else
            q2 = Q2;
            flag2 = 1;
        end
        
    case 2         %从1到0，流量缓慢减小
        if flag2 == 1
            t0_2 = t;
           flag2 = 0;
        end
        t1 = t - t0_2;
        
        if t1<=period
            q2 = Q2/period*(period - t1);
        else
            q2 = Q2;
            flag2 = 1;
        end
    otherwise
        q2 = Q2;
end

== matlab function VVA_pressure_dynamic_basefreq_sin/Q1 Q2/MATLAB Function3 ==
  data: Pout input; y output; Pin input
function y = fcn(Pout,Pin)

y=Pout/Pin;

== matlab function VVA_pressure_dynamic_basefreq_sin/VL ==
  data: P input; VL output; P0 input; Qm input
function VL= fcn(P,P0,Qm)


rou = 1.293*(P/P0); %密度，不考虑温度变化

VL=Qm*1000/rou ;

== matlab function VVA_pressure_dynamic_basefreq_sin/e ==
  data: P input; e output; Pr input; dP input; dPr input; de output
function [e,de]= fcn(P,Pr,dP,dPr)

e = Pr-P;
de=dPr-dP;

== matlab function VVA_pressure_dynamic_basefreq_sin/Q1 Q2/MATLAB Function2 ==
  data: Pout input; y output; Pin input
function y = fcn(Pout,Pin)

y=Pout/Pin;

== matlab function VVA_pressure_dynamic_basefreq_sin/MATLAB Function1 ==
  data: dm output; Q1 input; Q2 input; U1 input; U2 input
function dm = flow_calculate(Q1,Q2,U1,U2)

 dm =U1*Q1 -U2*Q2;

== matlab function VVA_pressure_dynamic_basefreq_sin/2阀模式 ==
  data: U1 output; U2 output; u input; action input
function [U1,U2] =ontrol(u,action)

switch (action)
    
    case 1       
        U1 = u;   %充气
        U2 = 0;

    case 2
        U1 = 0;   %不动
        U2 = 0;

    case 3    
        U1 = 0;   %放气
        U2 = u;
       
    otherwise
        U1 = 0;
        U2 = 0;    
end

== matlab function VVA_pressure_dynamic_basefreq_sin/dPL_dPR ==
  data: dP output size=1; T input; gamma input; Q input
function dP  = dP_fun(T,gamma,Q)

R=0.287;
V=1.57e-4;

dP = gamma*R*T*Q/V;

== matlab function VVA_pressure_dynamic_basefreq_sin/模式选择 ==
  data: e input; action output; et input
function action = control_test(e, et) %#codegen
% action: 1=充气, 2=不动, 3=放气
% 目标：减少抖动/省开关，但对正弦跟踪不引入过大滞后

Ts = 1e-4;            % 必须与你的 fixed-step 一致
Tmin = 0.003;         % 最小保持时间：建议 2~5ms 起步（这里 3ms）
Nmin = int32(Tmin/Ts);

% 滞回阈值（把进入阈值和退出阈值分开）
et_on  = et;          % 进入动作阈值
et_off = 0.6*et;      % 退出动作阈值（0.5~0.8*et 之间试）
et_big = 3.0*et;      % 逃逸阈值：误差很大时立即动作（2~5*et 之间试）

persistent a_prev hold_cnt
if isempty(a_prev)
    a_prev = int32(2);
    hold_cnt = int32(0);
end

% 计时器递减
if hold_cnt > 0
    hold_cnt = hold_cnt - 1;
end

% --- 施密特滞回决定“期望动作” ---
a_des = a_prev;

switch a_prev
    case 1  % 正在充气：除非误差回落到 et_off 内，否则保持充气
        if e <  et_off
            a_des = int32(2);
        else
            a_des = int32(1);
        end

    case 3  % 正在放气：除非误差回落到 -et_off 内，否则保持放气
        if e > -et_off
            a_des = int32(2);
        else
            a_des = int32(3);
        end

    otherwise % 当前不动：只有超过 et_on 才进入充/放
        if e >  et_on
            a_des = int32(1);
        elseif e < -et_on
            a_des = int32(3);
        else
            a_des = int32(2);
        end
end

% --- 逃逸条件：误差很大时不要被“最小保持”卡住 ---
escape = (abs(e) > et_big);

% --- 最小保持：只在“非逃逸”时生效 ---
if (hold_cnt > 0) && (~escape)
    action = a_prev;
else
    if a_des ~= a_prev
        hold_cnt = Nmin;     % 切换后启动保持窗口
    end
    action = a_des;
    a_prev = action;
end

end
